simulink model "PoursuiteSimu"  (R2017a)
settings: Solver=ode14x  StartTime=0.0  StopTime=70  FixedStep=0.001  RelTol=1e-3
values from neighbouring files (symbols this model uses):
  bornes = [minn, maxx]    [Model.m]
  K1 = cat(3,K1(1:r).sys)    [Mainscript.m]
  M = inv(X)    [Gainfind.m]    (also in GainfindV2.m; GainfindVTD.m; Mainscript.m = cat(3,M(1:r).sys); Observateurflou.m = inv(P))
  Parametres = [ax, bx, Rap, alpha, tau]    [Model.m]
  Parametres2 = [tr, f]    [Model.m]
settings Model: Creator=MONCEF  LastModifiedBy=MONCEF

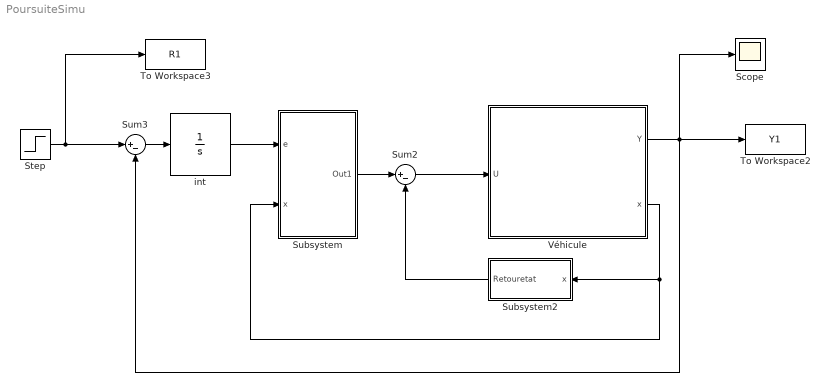
== system PoursuiteSimu ==
  Scope : Scope
  Step : Step  SampleTime=0
  Subsystem : Subsystem
  Subsystem2 : Subsystem
  Sum2 : Sum  Inputs=|+-
  Sum3 : Sum  Inputs=|+-
  To Workspace2 : ToWorkspace  VariableName=Y1  SaveFormat=Structure With Time  SampleTime=0.1
  To Workspace3 : ToWorkspace  VariableName=R1  SaveFormat=Structure With Time  SampleTime=0.1
  Véhicule : Subsystem
      mask Display: image(fullfile(pwd,'Images','VehiculeSuiveur.jpg'));
  int : Integrator
      mask Display: image(fullfile(pwd,'Images','Integrateur.png'));
  wires:
  int/1 -> Subsystem/1(e)
  Subsystem2/1(Retouretat) -> Sum2/2
  Véhicule/2(x) -> Subsystem/2(x), Subsystem2/1(x)
  Sum3/1 -> int/1
  Subsystem/1(Out1) -> Sum2/1
  Véhicule/1(Y) -> Scope/1, To Workspace2/1, Sum3/2
  Sum2/1 -> Véhicule/1(U)
  Step/1 -> To Workspace3/1, Sum3/1

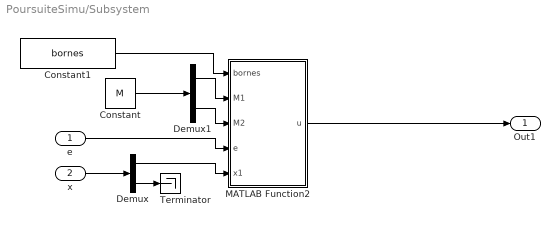
== system PoursuiteSimu/Subsystem ==
  e : Inport
  x : Inport  Port=2
  Constant : Constant  Value=M
  Constant1 : Constant  Value=bornes
  Demux : Demux  Outputs=2
  Demux1 : Demux  Outputs=2
  MATLAB Function2 : MATLAB Function  TreatAsAtomicUnit=on
  Terminator : Terminator
  Out1 : Outport
  wires:
  MATLAB Function2/1(u) -> Out1/1
  e/1 -> MATLAB Function2/4(e)
  x/1 -> Demux/1
  Demux/1 -> MATLAB Function2/5(x1)
  Demux/2 -> Terminator/1
  Constant/1 -> Demux1/1
  Demux1/1 -> MATLAB Function2/2(M1)
  Demux1/2 -> MATLAB Function2/3(M2)
  Constant1/1 -> MATLAB Function2/1(bornes)

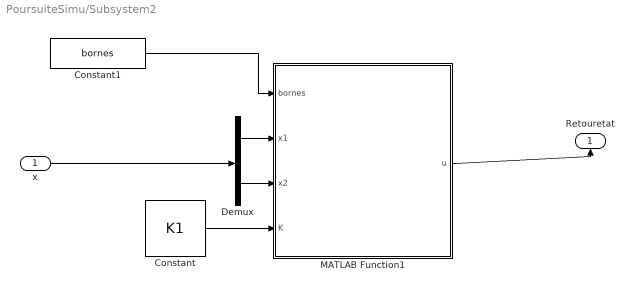
== system PoursuiteSimu/Subsystem2 ==
  x : Inport
  Constant : Constant  Value=K1
  Constant1 : Constant  Value=bornes
  Demux : Demux  Outputs=2
  MATLAB Function1 : MATLAB Function  TreatAsAtomicUnit=on
  Retouretat : Outport
  wires:
  Constant/1 -> MATLAB Function1/4(K)
  x/1 -> Demux/1
  Demux/2 -> MATLAB Function1/3(x2)
  Demux/1 -> MATLAB Function1/2(x1)
  MATLAB Function1/1(u) -> Retouretat/1
  Constant1/1 -> MATLAB Function1/1(bornes)

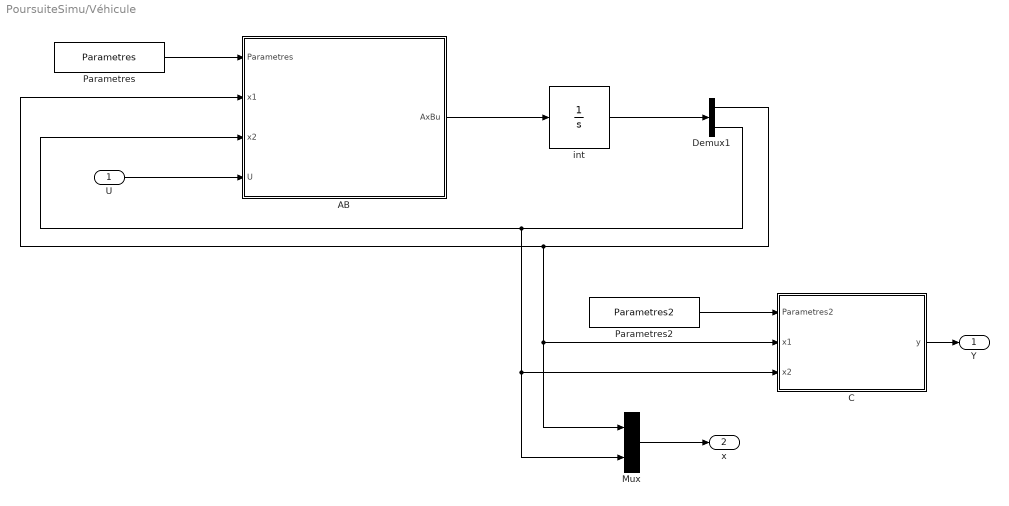
== system PoursuiteSimu/Véhicule ==
  U : Inport
  AB : MATLAB Function  TreatAsAtomicUnit=on
  C : MATLAB Function  TreatAsAtomicUnit=on
  Demux1 : Demux  Outputs=2
  Mux : Mux  Inputs=2
  Parametres : Constant  Value=Parametres
  Parametres2 : Constant  Value=Parametres2
  int : Integrator  InitialCondition=[0 0]
      mask Display: image(fullfile(pwd,'Images','Integrateur.png'));
  Y : Outport
  x : Outport  Port=2
  wires:
  C/1(y) -> Y/1
  Parametres/1 -> AB/1(Parametres)
  Parametres2/1 -> C/1(Parametres2)
  U/1 -> AB/4(U)
  AB/1(AxBu) -> int/1
  Demux1/2 -> Mux/2, C/3(x2), AB/3(x2)
  Demux1/1 -> Mux/1, C/2(x1), AB/2(x1)
  Mux/1 -> x/1
  int/1 -> Demux1/1

== matlab function PoursuiteSimu/Subsystem2/MATLAB Function1 ==
  data: bornes input; x1 input; x2 input; u output; K input
function u = fcn(bornes,x1,x2,K)

x=[x1;x2];

K1=K(:,:,1);
K2=K(:,:,2);

min = bornes(1);
max = bornes(2);
T1=(x1-min)/(max-min);
T2=(max-x1)/(max-min);



u =(T1*K1+T2*K2)*x;

== matlab function PoursuiteSimu/Subsystem/MATLAB Function2 ==
  data: bornes input; M1 input; M2 input; e input; u output; x1 input
function u = fcn(bornes,M1,M2,e,x1)

min = bornes(1);
max = bornes(2);
T1=(x1-min)/(max-min);
T2=(max-x1)/(max-min);

u =-(T1*M1+T2*M2)*e;

== matlab function PoursuiteSimu/Véhicule/AB ==
  data: Parametres input; x1 input; AxBu output; x2 input; U input
function AxBu = fcn(Parametres,x1,x2,U)

ax = Parametres(1);
bx = Parametres(2);
Rap = Parametres(3);
alpha = Parametres(4);
tau = Parametres(5);

%define the systeme matrix
A =[-(ax+bx*x1)/alpha Rap/alpha; 0 -1/tau];
B =[0 ; 1/tau];



AxBu = A*[x1;x2]+B*U;

== matlab function PoursuiteSimu/Véhicule/C ==
  data: Parametres2 input; x1 input; y output; x2 input
function y = fcn(Parametres2,x1,x2)
tr = Parametres2(1);
f = Parametres2(2);

C = [tr+f*x1 0];
y =C*[x1;x2];
